simulink model "quad_6D0F_ANSFT"  (R2023a)
settings: Solver=ode1  StartTime=0.0  StopTime=60  FixedStep=0.01  RelTol=1e-3
model workspace (MAT data in the model file):
  omega_n = 20
libraries: aerolibutil x1, simulink x1, robotcorelib x1, sharedtransform x1, uavutilslib x1
settings Model: Creator=Adan Daniel  LastModifiedBy=adan

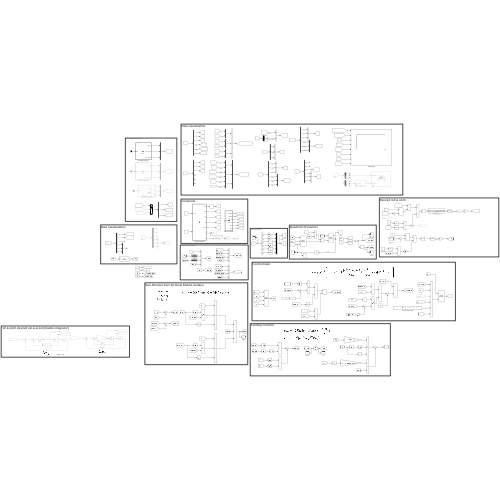
[thumbnail: Simulink's stored preview of the top-level diagram]
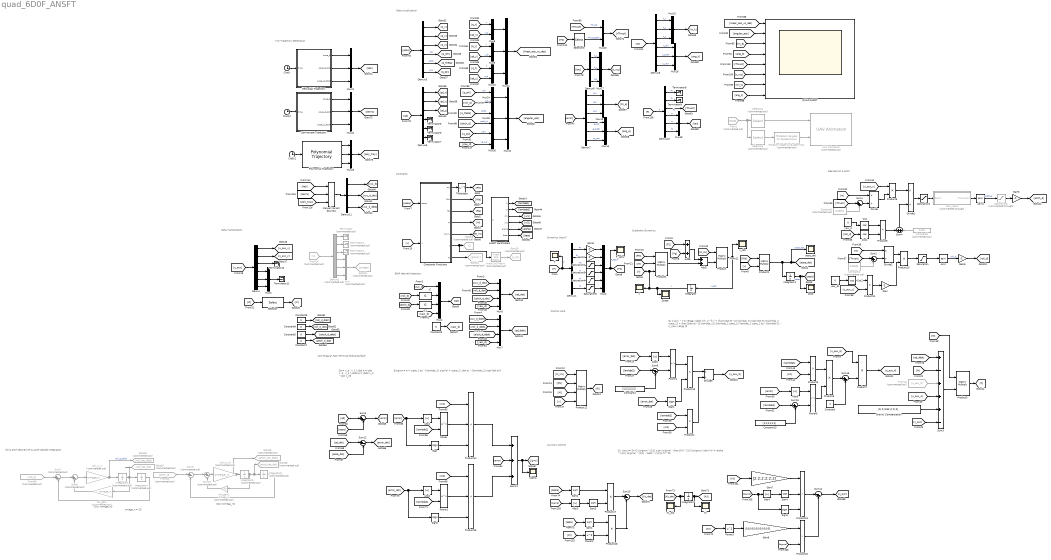
== system quad_6D0F_ANSFT ==
  note: omega_n = 20
  note: roll & pitch desired vel & accel [double integrator]
  note: Desired roll & pitch
  note: Quadrotor Dynamics
  note: XYZ Trajectory Generation
  note: Dynamics Input F
  note: $2\xi \omega_n$
  note: $2\xi \omega_n$
  note: 6DoF desired trajectory
  note: Constants
  note: Data manipulation
  note: Data visualization
  note: $e = x_d - x_1 \\ \dot e = \dot x_d - x_2 \\ \ddot e = \ddot x_d - \dot x_2$
  note: Non-Singular Fast Terminal Sliding Surface
  note: $\sigma = e + \zeta_1 |e| ^{\lambda_1} sign(e) + \zeta_2 | \dot e| ^{\lambda_2} sign(\dot e)$
  note: Auxiliary Control
  note: $u_{aux}=-2K(t) |\sigma|^{1/2} sign (\sigma) - \frac{K(t)^2}{2}\sigma \\ \dot K(t) = \alpha ^{1/2} |\sigma| ^{1/2} - \beta ^{1/2}K(t)^2$
  note: $u = g(x) ^{-1} \Bigg [ \ddot \chi_d - f(x) + \frac{|\dot e|^{2-\lambda_2} sign(\dot e)}{\lambda_2 \zeta_2} + \frac{|\dot e|^{2-\lambda_2}}{\lambda_2 \zeta_2} \lambda_1 \zeta_1 |e|^{\lambda-1} - u_{aux} \Bigg ]$
  note: Control Input
  ANSFT parameters : MATLAB Function  TreatAsAtomicUnit=on
  Abs{1..6} (6 alike) : Abs  SaturateOnIntegerOverflow=off
  Add2 : Sum
  Add5 : Sum
  Asin : Trigonometry  Operator=asin
  Asin1 : Trigonometry  Operator=asin
  Clock : Clock
  Clock1 : Clock
  Clock2 : Clock
  Constant : Constant
  Constant1 : Constant  Commented=on  Value=0.00001
  Constant10 : Constant  Value=[1;1;1;1;1;1]
  Constant2 : Constant  Commented=on  Value=0.00001
  Constant{3,5,7..9} (5 alike) : Constant  Value=0
  Constant4 : Constant  Value=[2;2;2;2;2;2]
  Constant6 : Constant  Commented=on  Value=0.001
  Constants Functions : MATLAB Function  TreatAsAtomicUnit=on
  Cos : Trigonometry  Operator=cos
  Cos1 : Trigonometry  Operator=cos
  Cos2 : Trigonometry  Operator=cos
  Demux{,1,5..8,10} (7 alike) : Demux  Outputs=6
  Demux11 : Demux  Outputs=3
  Demux2 : Demux  Commented=on  Outputs=6
  Demux9 : Demux  Outputs=3
  Divide{,1..3} (4 alike) : Product  Inputs=*/
  F : Scope
  F_satur : Scope
  From1 : From  Commented=on  GotoTag=pose
  From24 : From  Commented=on  GotoTag=v
  From42 : From  Commented=on  GotoTag=u_aux_3
  From60 : From  Commented=on  GotoTag=roll_d
  From61 : From  Commented=on  GotoTag=pitch_d
  Gain : Gain  Gain=-1
  Gain10 : Gain  Gain=0
  Gain5 : Gain  Gain=-1
  Gain6 : Gain  Gain=-1
  Gain7 : Gain  Gain=[2;2;2;2;2;2]
  Gain8 : Gain  Gain=[0.5;0.5;0.5;0.5;0.5;0.5]
  Gain9 : Gain  Gain=0
  Goto18 : Goto  Commented=on  GotoTag=J
  Goto19 : Goto  Commented=on  GotoTag=J_inv
  Goto20 : Goto  Commented=on  GotoTag=omega
  Goto31 : Goto  Commented=on  GotoTag=gravity
  Goto53 : Goto  Commented=on  GotoTag=roll_hat_ddot
  Goto54 : Goto  Commented=on  GotoTag=roll_hat_dot
  Goto55 : Goto  Commented=on  GotoTag=pitch_hat_ddot
  Goto56 : Goto  Commented=on  GotoTag=pitch_hat_dot
  Gravity Compensation : Constant  Value=[0; 0; 9.81; 0; 0; 0]
  Helicoidal Trajectory : MATLAB Function  TreatAsAtomicUnit=on
  IC : InitialCondition  Value=0
  IC1 : InitialCondition  Value=0
  Integrator : Integrator  InitialCondition=[0; 0; 0; 0; 0; 0]
  Integrator1 : Integrator  InitialCondition=[0; 0; 0; 0; 0; 0]
  Integrator{2,4..6} (4 alike) : Integrator  Commented=on
  Integrator7 : Integrator  InitialCondition=[0;0;0;0;0;0]
  Invert 3x3 Matrix : aerolibutil/Invert  3x3 Matrix  Commented=on
  Kt : Scope
  Kt_dot : Scope
  Lemniscate Trajectory : MATLAB Function  TreatAsAtomicUnit=on
  Manual Variant Source1 : simulink/Signal Routing/Manual Variant Source  NumChoices=3  LabelModeActiveChoice=V_1
  Mux : Mux  Commented=on  Inputs=3
  Mux{8..10,20,24..26} (7 alike) : Mux  Inputs=2
  Mux{3,11..18,21..23} (12 alike) : Mux  Inputs=3
  Mux2 : Mux  Inputs=6
  Mux4 : Mux
  Mux6 : Mux
  Mux7 : Mux
  Polynomial Trajectory : robotcorelib/Polynomial Trajectory  WaypointSource=Internal  Waypoints=[0, 0, 0, 0, 0, 0; 0, 0, 0, 0, 0, 0; 0, 2, 5, 2, 5, 2]  TimePoints=[ 0, 12, 24, 36, 48, 60]  TimeInterval=[ 1, 4 ]  Method=Cubic Polynomial  ParameterSource=Internal  VelocityBoundaryCondition=zeros( 3, 6)  AccelerationBoundaryCondition=zeros( 2, 5 )  SimulateUsing=Interpreted execution
  Power{,1,4..5} (4 alike) : Math  Operator=pow
  Power2 : Math  Operator=square
  Power3 : Math  Operator=square
  Product : Product  Multiplication=Matrix(*)
  Product1 : Product  Inputs=3  Multiplication=Matrix(*)
  Product{4..11,13,16..18} (12 alike) : Product
  Product12 : Product  Inputs=4  Multiplication=Matrix(*)
  Product14 : Product  Inputs=3
  Product15 : Product  Inputs=3
  Product19 : Product  Inputs=3
  Product2 : Product  Multiplication=Matrix(*)
  Product3 : Product  Multiplication=Matrix(*)
  QUAD ANSFT : Scope  NumInputPorts=8
  Rotation Angles to Quaternions : sharedtransform/Rotation Angles to Quaternions  Commented=on  rotationOrder=ZYX  aMode=aMode
  Saturation : Saturate  UpperLimit=1  LowerLimit=-1
  Saturation1 : Saturate  UpperLimit=1  LowerLimit=-1
  Saturation2 : Saturate  UpperLimit=5.8*4  LowerLimit=0
  Saturation3 : Saturate
  Saturation4 : Saturate
  Saturation5 : Saturate
  Saturation6 : Saturate  Commented=through  UpperLimit=0.1  LowerLimit=-0.1
  Scope : Scope
  Selector : Selector  NumberOfDimensions=2  InputPortWidth=3  IndexOptions=Index vector (dialog),Index vector (dialog)  Indices=1,1  OutputSizes=1,1
  Selector3 : Selector  InputPortWidth=6  IndexOptions=Index vector (dialog)  Indices=[3]  OutputSizes=1
  Selector4 : Selector  Commented=on  InputPortWidth=6  IndexOptions=Index vector (dialog)  Indices=[1 2 3]  OutputSizes=1
  Selector5 : Selector  Commented=on  InputPortWidth=6  IndexOptions=Index vector (dialog)  Indices=[6 5 4]  OutputSizes=1
  Sign{,1..3} (4 alike) : Signum
  Sqrt{1..4} (4 alike) : Sqrt
  Sum1 : Sum  Inputs=|++
  Sum{7..10} (4 alike) : Sum  Commented=on  Inputs=|+-
  Sum11 : Sum  Inputs=+++
  Sum{5,12..13,15} (4 alike) : Sum  Inputs=|+-
  Sum14 : Sum  Inputs=|--
  Sum16 : Sum  Inputs=|++
  Sum2 : Sum  Inputs=|++
  Sum3 : Sum  Inputs=+-+++-
  Sum4 : Sum
  Sum6 : Sum  Inputs=|-+
  Terminator : Terminator  Commented=on
  Terminator1 : Terminator  Commented=on
  Terminator{5..11} (7 alike) : Terminator
  Terminator2 : Terminator  Commented=on
  Transpose : Math  Operator=transpose
  UAV Animation : uavutilslib/UAV Animation  Commented=on  UAVType=Multirotor  UAVSize=1  InertialZDirection=Up  SampleTime=-1
  asin_satur : MATLAB Function  Commented=through  TreatAsAtomicUnit=on
  pose : Scope
  pose_dot : Scope
  roll_gain : Gain  Commented=on  Gain=omega_n
  roll_gain1 : Gain  Commented=on  Gain=omega_n
  roll_w_n : Gain  Commented=on  Gain=omega_n
  roll_w_n1 : Gain  Commented=on  Gain=omega_n
  sigma : Scope
  v : Scope
  v_dot : Scope
  yaw_d : Constant  Value=0
  yaw_d1 : Constant  Value=0
  wires:
  [v] -> Product2/2
  Product2/1 -> Integrator1/1, pose_dot/1, [pose_dot]  "pose_dot"
  Product/1 -> v_dot/1, Integrator/1  "v_dot"
  Integrator1/1 -> pose/1, [pose]  "pose"
  Integrator/1 -> Scope/1, v/1, [v], Product1/3  "v"
  Add5/1 -> Add2/1
  [M] -> Product1/2
  [Fg] -> Add5/2
  Add2/1 -> Product/2
  [Rib] -> Product2/1
  [Phi] -> Product1/1
  Product1/1 -> Add2/2
  [F2] -> Add5/1
  [M_inv] -> Product/1
  [pose] -> Constants Functions/1(pose)
  [v] -> Constants Functions/2(v)
  Constants Functions/1(Phi) -> Transpose/1
  Constants Functions/4(M) -> [M]
  Constants Functions/3(Fg) -> [Fg]
  Constants Functions/5(M_inv) -> [M_inv]
  Constants Functions/2(Rib) -> [Rib]
  Transpose/1 -> [Phi]
  Clock1/1 -> Polynomial Trajectory/1
  Saturation5/1 -> Mux2/6
  Demux1/5 -> Saturation4/1  "ty"
  Saturation3/1 -> Mux2/4
  Saturation2/1 -> Mux2/3
  Demux1/1 -> Gain9/1  "Fx"
  Demux1/2 -> Gain10/1  "Fy"
  Mux2/1 -> F_satur/1, [F2]  "F_satur"
  [F] -> F/1, Demux1/1  "F"
  Saturation4/1 -> Mux2/5
  Demux1/6 -> Saturation5/1  "tz"
  Demux1/4 -> Saturation3/1  "tx"
  Demux1/3 -> Saturation2/1  "Fz"
  ANSFT parameters/5(alpha) -> [alpha]
  ANSFT parameters/2(lambda2) -> [lambda2]
  ANSFT parameters/3(xi1) -> [xi1]
  ANSFT parameters/4(xi2) -> [xi2]
  ANSFT parameters/1(lambda1) -> [lambda1]
  [u_aux] -> Demux/1
  Demux/1 -> [u_aux_x]
  Demux/2 -> [u_aux_y]
  Constants Functions/6(J) -> Invert 3x3 Matrix/1, Goto18/1
  Mux3/1 -> Terminator11/1
  Demux/4 -> Mux3/1
  Demux/6 -> Mux3/3
  Demux/5 -> Mux3/2
  [M] -> Selector/1
  Selector/1 -> [m]
  Constant3/1 -> [yaw_d]
  [yaw_d] -> Mux4/4
  [xyz_d] -> Mux4/1
  Mux4/1 -> [qd]
  Demux/3 -> Terminator10/1
  Divide1/1 -> Saturation1/1
  [u_aux_y] -> Product11/2
  Cos1/1 -> Product9/2
  [m] -> Divide2/1
  Sum1/1 -> Divide/2
  Gain/1 -> Product10/2
  [Thrust] -> Sum2/1
  yaw_d1/1 -> Cos2/1
  Constant1/1 -> Sum1/2
  Product11/1 -> Gain/1
  Cos/1 -> Product9/1
  Product10/1 -> Saturation/1
  Constant2/1 -> Sum2/2
  [roll_d] -> Cos1/1
  Divide2/1 -> Product10/1
  Divide/1 -> Product8/2
  Sum2/1 -> Divide2/2
  [u_aux_x] -> Product8/1
  Cos2/1 -> Product11/1
  Asin1/1 -> Saturation6/1  "pitch_d"
  [Thrust] -> Sum1/1
  Saturation/1 -> Asin/1
  Saturation1/1 -> asin_satur/1(param)
  yaw_d/1 -> Cos/1
  Product8/1 -> Divide1/1
  [m] -> Divide/1
  Asin/1 -> Gain6/1  "roll_d"
  Sum7/1 -> Sum8/1
  From60/1 -> Sum7/1
  Integrator2/1 -> Goto54/1, Integrator4/1, roll_gain/1
  roll_gain/1 -> Sum8/2
  Integrator6/1 -> Sum9/2
  Sum9/1 -> Sum10/1
  Sum8/1 -> roll_w_n/1
  Integrator4/1 -> Sum7/2
  Integrator5/1 -> roll_gain1/1, Goto56/1, Integrator6/1
  roll_w_n/1 -> Integrator2/1, Goto53/1  "roll_d_ddot"
  roll_w_n1/1 -> Goto55/1, Integrator5/1
  roll_gain1/1 -> Sum10/2
  From61/1 -> Sum9/1
  Sum10/1 -> roll_w_n1/1
  [yaw_d] -> Mux6/4
  [roll_d_dot] -> Mux6/2
  [xyz_d_dot] -> Mux6/1
  [pitch_d_dot] -> Mux6/3
  Mux6/1 -> [qd_dot]
  [yaw_d] -> Mux7/4
  [roll_d_ddot] -> Mux7/2
  [xyz_d_ddot] -> Mux7/1
  [pitch_d_ddot] -> Mux7/3
  Mux7/1 -> [qd_ddot]
  Product9/1 -> Sum4/1
  Sum4/1 -> Divide1/2
  Constant6/1 -> Sum4/2
  Demux2/1 -> Terminator/1
  Mux/1 -> Goto20/1
  Demux2/3 -> Terminator2/1
  Demux2/4 -> Mux/1
  Demux2/5 -> Mux/2
  From24/1 -> Demux2/1
  Demux2/6 -> Mux/3
  Demux2/2 -> Terminator1/1
  Constants Functions/7(g) -> Goto31/1
  IC/1 -> Mux4/2
  [roll_d] -> IC/1
  IC1/1 -> Mux4/3
  [pitch_d] -> IC1/1
  Invert 3x3 Matrix/1 -> Goto19/1
  [pose] -> Demux5/1
  Demux5/1 -> [q_x]
  Demux5/2 -> [q_y]
  Demux5/3 -> [q_z]
  Demux5/6 -> [q_psi]  "yaw"
  Demux5/4 -> [q_phi]  "roll"
  Demux5/5 -> [q_theta]  "pitch"
  Demux6/1 -> [qd_x]
  Demux6/2 -> [qd_y]
  [qd] -> Demux6/1
  Demux6/6 -> Terminator7/1
  Demux6/3 -> [qd_z]
  Demux6/5 -> Terminator6/1
  Demux6/4 -> Terminator5/1
  [q_x] -> Mux8/1  "x"
  [qd_x] -> Mux8/2  "x_d"
  [q_y] -> Mux9/1  "y"
  [qd_y] -> Mux9/2  "y_d"
  [q_z] -> Mux10/1  "z"
  [qd_z] -> Mux10/2  "z_d"
  Mux10/1 -> Mux11/3
  Mux9/1 -> Mux11/2
  Mux8/1 -> Mux11/1
  Mux11/1 -> [linear_pos_vs_des]
  [linear_pos_vs_des] -> QUAD ANSFT/1
  Mux12/1 -> [angular_pos]
  [error] -> Demux7/1
  Demux7/3 -> Mux13/3  "e_z"
  Demux7/2 -> Mux13/2  "e_y"
  Demux7/1 -> Mux13/1  "e_x"
  Demux7/6 -> Mux14/3  "e_yaw"
  Demux7/4 -> Mux14/1  "e_roll"
  Demux7/5 -> Mux14/2  "e_pitch"
  Mux13/1 -> [lin_e]
  Mux14/1 -> [ang_e]
  Mux15/1 -> [lin_k]
  Demux8/6 -> Mux16/3  "k_yaw"
  [Kt] -> Demux8/1
  Demux8/2 -> Mux15/2  "k_y"
  Demux8/4 -> Mux16/1  "k_roll"
  Demux8/3 -> Mux15/3  "k_z"
  Demux8/1 -> Mux15/1  "k_x"
  Demux8/5 -> Mux16/2  "k_pitch"
  Mux16/1 -> [ang_k]
  [ang_k] -> QUAD ANSFT/8
  [angular_pos] -> QUAD ANSFT/2
  [lin_e] -> QUAD ANSFT/3
  [ang_e] -> QUAD ANSFT/4
  [lin_k] -> QUAD ANSFT/7
  Constant5/1 -> [pitch_d_ddot]
  Constant7/1 -> [pitch_d_dot]
  Constant9/1 -> [roll_d_dot]
  Constant8/1 -> [roll_d_ddot]
  Saturation6/1 -> Gain5/1
  asin_satur/1(final_param) -> Asin1/1
  Gain5/1 -> [pitch_d]
  Gain6/1 -> [roll_d]
  [tau] -> Demux9/1
  Demux9/1 -> Mux17/1  "t_x"
  Demux9/3 -> Mux17/3  "t_z"
  Demux9/2 -> Mux17/2  "t_y"
  Mux17/1 -> [t_xyz]
  [t_xyz] -> QUAD ANSFT/6
  [F2] -> Selector3/1
  [Thrust] -> Mux20/1  "Thrust"
  Selector3/1 -> Mux20/2  "Thrust_satur"
  Mux20/1 -> [rThrust]
  [rThrust] -> QUAD ANSFT/5
  Mux22/1 -> [lemni]
  Clock/1 -> Helicoidal Trajectory/1(time)
  Lemniscate Trajectory/3(pose_d_ddot) -> Mux22/3
  Helicoidal Trajectory/3(pose_d_ddot) -> Mux21/3
  Clock2/1 -> Lemniscate Trajectory/1(time)
  Lemniscate Trajectory/2(pose_d_dot) -> Mux22/2
  Helicoidal Trajectory/1(pose_d) -> Mux21/1
  Lemniscate Trajectory/1(pose_d) -> Mux22/1
  Helicoidal Trajectory/2(pose_d_dot) -> Mux21/2
  Mux21/1 -> [heli]
  Demux11/1 -> [xyz_d]
  Demux11/3 -> [xyz_d_ddot]
  Demux11/2 -> [xyz_d_dot]
  Manual Variant Source1/1 -> Demux11/1
  Polynomial Trajectory/1 -> Mux23/1
  Polynomial Trajectory/3 -> Mux23/3
  Polynomial Trajectory/2 -> Mux23/2
  Mux23/1 -> [poly_tray]
  [heli] -> Manual Variant Source1/1
  [poly_tray] -> Manual Variant Source1/3
  [lemni] -> Manual Variant Source1/2
  [q_phi] -> Mux24/1  "roll"
  [roll_d] -> Mux24/2  "roll_d"
  [pitch_d] -> Mux25/2  "pitch_d"
  [q_theta] -> Mux25/1  "pitch"
  Mux24/1 -> Mux12/1
  Mux25/1 -> Mux12/2
  [q_psi] -> Mux26/1  "yaw"
  [yaw_d] -> Mux26/2  "yaw_d"
  Mux26/1 -> Mux12/3
  Power1/1 -> Product15/2
  Power/1 -> Product14/2
  Product15/1 -> Sum11/3
  Sum5/1 -> [error]
  Sign2/1 -> Product15/3
  [error] -> Sign/1, Abs1/1
  Sum12/1 -> [error_dot]
  Abs1/1 -> Power/1
  [error] -> Sum11/2
  [xi1] -> Product14/1
  [error_dot] -> Sign2/1, Abs2/1
  [lambda1] -> Power/2
  [lambda2] -> Power1/2
  Product14/1 -> Sum11/1
  [qd_dot] -> Sum12/1
  [qd] -> Sum5/1
  [pose] -> Sum5/2
  Sign/1 -> Product14/3
  Sum11/1 -> sigma/1, [sigma]
  [pose_dot] -> Sum12/2
  [xi2] -> Product15/1
  Abs2/1 -> Power1/1
  Power3/1 -> Gain8/1
  Sqrt1/1 -> Product18/1
  Abs3/1 -> Sqrt3/1
  Sign3/1 -> Product19/3
  [Kt] -> Gain7/1
  Product19/1 -> Sum14/1
  Product18/1 -> Sum13/2
  Sqrt4/1 -> Product19/2
  [Kt] -> Power3/1
  Integrator7/1 -> Kt/1, [Kt]
  Sum13/1 -> [Kt_dot]
  Sqrt2/1 -> Product17/1
  Product16/1 -> Sum14/2
  [alpha] -> Sqrt2/1
  [sigma] -> Product16/2
  [sigma] -> Abs3/1
  Gain7/1 -> Product19/1
  [beta] -> Sqrt1/1
  [sigma] -> Sign3/1, Abs4/1
  Sum14/1 -> [u_aux]
  [Kt_dot] -> Kt_dot/1, Integrator7/1
  [Kt] -> Power2/1
  Product17/1 -> Sum13/1
  Gain8/1 -> Product16/1
  Power2/1 -> Product18/2
  Abs4/1 -> Sqrt4/1
  Sqrt3/1 -> Product17/2
  ANSFT parameters/6(beta) -> [beta]
  Demux10/1 -> Terminator8/1  "Fx"
  Demux10/2 -> Terminator9/1  "Fy"
  Demux10/5 -> Mux18/2  "ty"
  Demux10/4 -> Mux18/1  "tx"
  [F] -> Demux10/1  "F"
  Demux10/3 -> [Thrust]  "Fz"
  Demux10/6 -> Mux18/3  "tz"
  Mux18/1 -> [tau]
  Gain9/1 -> Mux2/1
  Gain10/1 -> Mux2/2
  Selector4/1 -> UAV Animation/1
  Selector5/1 -> Rotation Angles to Quaternions/1
  From1/1 -> Selector5/1, Selector4/1
  Rotation Angles to Quaternions/1 -> UAV Animation/2
  Sign1/1 -> Product13/2
  Product6/1 -> Sum16/1
  [error] -> Abs6/1
  [error_dot] -> Sign1/1
  [error_dot] -> Abs5/1
  [u_aux] -> Sum3/6
  Sum16/1 -> Product7/2
  Constant4/1 -> Sum6/2
  Constant10/1 -> Sum15/2
  [Phi] -> Product12/2
  [fx] -> Sum3/2
  Power5/1 -> Product6/2
  Sum3/1 -> Product3/2
  Constant/1 -> Sum16/2
  [M] -> Product12/3
  [M_inv] -> Product12/1
  Product4/1 -> Divide3/2
  Product3/1 -> [F]
  [xi1] -> Product5/2
  [u_aux_4] -> Sum3/4
  [M] -> Product3/1
  [lambda2] -> Product4/1
  Sum15/1 -> Power5/2
  [lambda1] -> Product5/1
  Product5/1 -> Product6/1
  Product12/1 -> [fx]
  [qd_ddot] -> Sum3/1
  Divide3/1 -> [u_aux_3]
  Product7/1 -> [u_aux_4]
  Gravity Compensation/1 -> Sum3/5
  [lambda1] -> Sum15/1
  From42/1 -> Sum3/3
  Abs5/1 -> Power4/1
  Sum6/1 -> Power4/2
  [u_aux_3] -> Product7/1
  Power4/1 -> Product13/1
  [xi2] -> Product4/2
  Product13/1 -> Divide3/1
  [v] -> Product12/4
  [lambda2] -> Sum6/1
  Abs6/1 -> Power5/1

== matlab function quad_6D0F_ANSFT/ANSFT parameters ==
  data: lambda1 output; unused input; lambda2 output; xi1 output; xi2 output; alpha output; beta output
function [lambda1, lambda2, xi1, xi2, alpha, beta]= fcn(~)

xi1 = [1; 1; 0.01; 8; 8; 5];

xi2 = [13; 13; 2; 0.5; 0.5; 0.5];
% bets
lambda1 = [2; 2; 2; 5; 5; 5];

lambda2 = [1.3; 1.3; 1.3; 1.3; 1.3; 1.3];

alpha = [0.005; 0.005; 0.05; 10; 10; 20];

beta = [15; 15; 5; 0.005; 0.005; 5];

== matlab function quad_6D0F_ANSFT/asin_satur ==
  data: param input; final_param output
function final_param = asin_saturation(param)

if param > 1
    final_param = 1;
elseif param < -1
    final_param = -1;
else
    final_param = param;
end

== matlab function quad_6D0F_ANSFT/Constants Functions ==
  data: Phi output; Rib output; Fg output; pose input; M output; M_inv output; v input; J output; g output
function [Phi, Rib, Fg, M, M_inv, J, g]   = fcn(pose, v)

%% System constants
m = 2; %5 mass 2.2 kg
l = 0.25; % m
g = 9.81; % gravity
Jxx =  0.0411; % kg m²
Jyy = 0.0478; % kg m²
Jzz = 0.0599; % kg m²
kT = 3.4e-5;
kQ = 3.4e-6;
%% Phi vector 6d

uu = v(1);
vv = v(2);
ww = v(3);
pp = v(4);
qq = v(5);
rr = v(6);


Phi = [0, -rr, qq, 0, -ww, vv;
        rr, 0, -pp , ww, 0, -uu;
        -qq, pp, 0,  -vv, uu, 0;
        0, 0, 0, 0, -rr, qq; 
        0, 0, 0, rr, 0, -pp;
        0, 0, 0, -qq, pp, 0];
%% Fg and Rib calculation

roll = pose(4);
pitch = pose(5);
yaw = pose(6);


Rib = [cos(yaw)*cos(pitch), -cos(roll)*sin(yaw) + cos(yaw)*sin(roll)*sin(pitch), sin(roll)*sin(yaw) + cos(roll)*cos(yaw)*sin(pitch), 0, 0, 0;
       cos(pitch)*sin(yaw), cos(roll)*cos(yaw) + sin(yaw)*sin(pitch)*sin(roll), -cos(yaw)*sin(roll) + sin(yaw)*sin(pitch)*cos(roll), 0, 0, 0;
       -sin(pitch), cos(pitch)*sin(roll), cos(pitch)*cos(roll), 0, 0, 0;
       0, 0, 0, 1, sin(roll)*tan(pitch), cos(roll)*tan(pitch);
       0, 0, 0, 0, cos(roll), -sin(roll);
       0, 0, 0, 0, sin(roll)/cos(pitch), cos(roll)/cos(pitch)];

Fg = [m*g*sin(pitch);
      -m*g*cos(pitch)*sin(roll);
      -m*g*cos(pitch)*cos(roll);
      0;
      0;
      0];

%% M matrix

M = [m, 0, 0, 0, 0, 0;
    0, m, 0, 0, 0, 0;
    0, 0, m, 0, 0, 0;
    0, 0, 0, Jxx, 0, 0;
    0, 0, 0, 0, Jyy, 0;
    0, 0, 0, 0, 0, Jzz];

M_inv = inv(M);

%% Allocation matrix

% allo = [0, 0, 0, 0, 0, 0;
%         0, 0, 0, 0, 0, 0;
%         kT, kT, kT, kT, kT, kT;
%         -kT*l, kT*l, kT*l/2, -kT*l/2, -kT*l/2, kT*l/2;
%         0, 0, -sqrt(3)*kT*l/2, sqrt(3)*kT*l/2, -sqrt(3)*kT*l/2, sqrt(3)*kT*l/2;
%         kQ, -kQ, kQ, -kQ, -kQ, kQ,];
% 
% allo = pinv(allo);

J = [Jxx, 0, 0;
     0, Jyy, 0;
     0, 0, Jzz];

== matlab function quad_6D0F_ANSFT/Helicoidal Trajectory ==
  data: time input; pose_d output; pose_d_dot output; pose_d_ddot output
function [pose_d, pose_d_dot, pose_d_ddot]= fcn(time)

pos_z = time / 12;
f = 0.15;
arg = f * (time - 5);
r = 2;

% hover for 5 s | include inclination in roll
% 5 metros al menos

if (time < 5)
    pos_x = 0;
    pos_y = 0;
    % roll = 0;
else
    pos_x = - 2 + r * cos (arg);
    pos_y = r * sin (arg);
    % roll = 0.15;
end

% roll = 0;
% yaw = time * 0;

pose_d = [pos_x;
          pos_y;
          pos_z];
          % roll;
          % 0;
          % yaw];

pos_z_dot = 1 / 12;

% hover for 5 s
if (time < 5)
    pos_x_dot = 0;
    pos_y_dot = 0;
else
    pos_x_dot = - f * r * sin(arg);
    pos_y_dot = f * r * cos(arg);
end

% yaw_dot = 0;

pose_d_dot = [pos_x_dot;
              pos_y_dot;
              pos_z_dot];
              % 0;
              % 0;
              % yaw_dot];

pos_z_ddot = 0;
% hover for 5 s
if (time < 5)
    pos_x_ddot = 0;
    pos_y_ddot = 0;
else
    pos_x_ddot = - f * f * r * cos(arg);
    pos_y_ddot = - f * f * r * sin(arg);
end

% yaw_ddot = 0;

pose_d_ddot = [pos_x_ddot;
               pos_y_ddot;
               pos_z_ddot];
               % 0;
               % 0;
               % yaw_ddot];

== matlab function quad_6D0F_ANSFT/Lemniscate Trajectory ==
  data: time input; pose_d output; pose_d_dot output; pose_d_ddot output
function [pose_d, pose_d_dot, pose_d_ddot]= fcn(time)

%% Positions

arg = time / 4;

pos_x = cos(arg) ./ (1 + sin(arg) .* sin(arg));
pos_y = cos(arg) .* sin(arg) ./ (1 + sin(arg) .* sin(arg));
pos_z = sin(arg);

% yaw = time * 0;

pose_d = [pos_x;
          pos_y;
          pos_z];
          % 0;
          % 0;
          % yaw];

%% Velocities

pos_z_dot = 0.25 * cos(arg);
pos_x_dot = - sin(arg)/(4*(sin(arg)^2 + 1)) - (cos(arg)^2*sin(arg))/(2*(sin(arg)^2 + 1)^2);
pos_y_dot = cos(arg)^2/(4*(sin(arg)^2 + 1)) - sin(arg)^2/(4*(sin(arg)^2 + 1)) - (cos(arg)^2*sin(arg)^2)/(2*(sin(arg)^2 + 1)^2);
% yaw_dot = 0;

pose_d_dot = [pos_x_dot;
              pos_y_dot;
              pos_z_dot];
              % 0;
              % 0;
              % yaw_dot];

%% Accelerations

pos_z_ddot = -0.25 * 0.25 * sin(arg);
pos_x_ddot = 0;
pos_y_ddot = 0;
% yaw_ddot = 0;

pose_d_ddot = [pos_x_ddot;
               pos_y_ddot;
               pos_z_ddot];
               % 0;
               % 0;
               % yaw_ddot];
